simulink model "Bixler_withAutoPilot"  (R2018b)
settings: Solver=FixedStepAuto  StartTime=0.0  StopTime=inf  RelTol=1e-3
undefined symbols (not defined in the file or in its folder): dev, Main, pwm_output0
libraries: simulink x5, px4uORBlib x4, aerolibutil x3, px4Sensorslib x2, vrlib x1, px4lib x1, sharedtransform x1
(part 1 of 2)
settings Model: SimulationMode=external  ExtModeTrigDuration=10  Creator=Robert  LastModifiedBy=Robert
settings SolverCC: PositivePriorityOrder=on
settings DataIOCC: SaveState=on
settings OptimizationCC: DefaultUnderspecifiedDataType=single  EnhancedBackFolding=on  PassReuseOutputArgsAs=Individual arguments  MaxStackSize=64  OptimizeBlockOrder=speed  DifferentSizesBufferReuse=on  OptimizationCustomize=off
settings DebuggingCC: ParameterTunabilityLossMsg=error
settings HardwareCC: ProdBitPerPointer=32  ProdBitPerSizeT=32  ProdBitPerPtrDiffT=32  ProdLargestAtomicInteger=Long  ProdLargestAtomicFloat=Double  ProdWordSize=32  ProdLongLongMode=on  ProdHWDeviceType=ARM Compatible->ARM Cortex
settings SFSimCC: MATLABDynamicMemAlloc=off
settings RTWCC: SystemTargetFile=ert.tlc  HardwareBoard=PX4 Pixhawk 1  TLCOptions="-aInlineSetEventsForThisBaseRateFcn=TLC_FALSE -aSuppressMultiTaskScheduler=TLC_FALSE  -aRateBasedStepFcn=0"  TemplateMakefile=ert_default_tmf  GenerateReport=on  Toolchain=GNU Tools for PX4 Autopilots  IncludeHyperlinkInReport=on  LaunchReport=on  TargetLang=C++  GenerateTraceInfo=on  GenerateTraceReport=on  GenerateTraceReportSl=on  GenerateTraceReportSf=on  GenerateTraceReportEml=on
settings CodeAppCC: ForceParamTrailComments=on  IgnoreCustomStorageClasses=off  OperatorAnnotations=on  SimulinkDataObjDesc=on  SFDataObjDesc=on  InsertBlockDesc=on
settings ERTTargetCC: ExtMode=on  ExtModeMexArgs='127.0.0.1' 1 17725

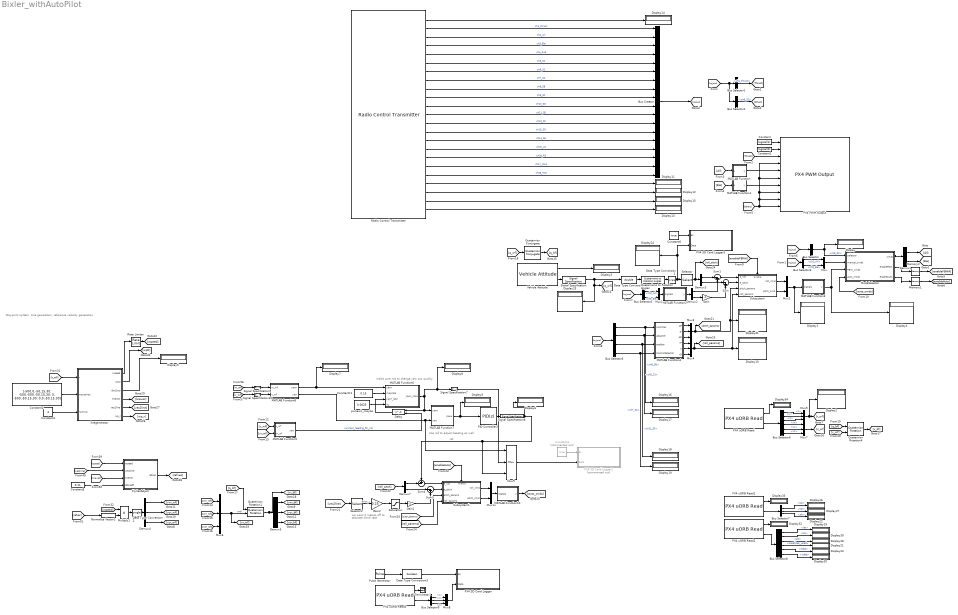
== system Bixler_withAutoPilot ==
  note: we want 4 metres off
      | to saturate climb rate
  note: Waypoint system,
      | Line generation,
      | reference velocity generation
  note: make sure not to change yaw too quickly
  note: Use roll to adjust heading as well
  Bus Creator : BusCreator  Inputs=18
  Bus Selector : BusSelector  OutputSignals=ch9_SC
  Bus Selector1 : BusSelector  OutputSignals=ch1_thrust
  Bus Selector2 : BusSelector  OutputSignals=ch6_S2
  Bus Selector3 : BusSelector  OutputSignals=ch2_Ail,ch3_Ele
  Bus Selector4 : BusSelector  OutputSignals=ch2_Ail,ch3_Ele
  Bus Selector5 : BusSelector  OutputSignals=ch8_SB,ch5_S1,ch12_SF,ch7_SA
  Bus Selector6 : BusSelector  OutputSignals=x,y,z,vx,vy,vz
  Bus Selector7 : BusSelector  OutputSignals=lat,lon,alt
  Bus Selector8 : BusSelector  OutputSignals=lat,lon,alt,satellites_used,hdop,vdop
  Bus Selector9 : BusSelector  OutputSignals=x,y,z
  Constant : Constant  Value=logical(1)
  Constant1 : Constant  Value=logical(0)
  Constant11 : Constant  Value=0.15  OutDataTypeStr=single
  Constant2 : Constant  Value=[-500,0,-50,15,30; -500,-500,-50,15,30; 0, -500,-50,15,30; 0,0,-50,15,30]  OutDataTypeStr=single
  Constant3 : Constant  Value=4  OutDataTypeStr=single
  Constant4 : Constant  Commented=on  Value=true  OutDataTypeStr=boolean
  Constant5 : Constant  Value=0.11  OutDataTypeStr=single  SampleTime=-1
  Constant6 : Constant  Value=true  OutDataTypeStr=boolean
  Data Type Conversion : DataTypeConversion  OutDataTypeStr=double
  Data Type Conversion1 : DataTypeConversion  OutDataTypeStr=single
  Data Type Conversion2 : DataTypeConversion  OutDataTypeStr=single
  Data Type Conversion3 : DataTypeConversion  OutDataTypeStr=boolean
  Delay : Delay  DelayLength=1  InitialConditionSource=Input port
      settings: InputPortMap=u0,p4
  Demux{1..3,7} (4 alike) : Demux  Outputs=2
  Demux4 : Demux  Outputs=3
  Demux5 : Demux  Outputs=3
  Display{,1..34} (35 alike) : Display
  FlyVecAdjust : MATLAB Function  TreatAsAtomicUnit=on
  Gain : Gain  Gain=-1
  Gain1 : Gain  Gain=-1
  Gain2 : Gain  Gain=0.25
  MATLAB Function : MATLAB Function  TreatAsAtomicUnit=on
  MATLAB Function1 : MATLAB Function  TreatAsAtomicUnit=on
  MATLAB Function10 : MATLAB Function  TreatAsAtomicUnit=on
  MATLAB Function2 : MATLAB Function  TreatAsAtomicUnit=on
  MATLAB Function3 : MATLAB Function  TreatAsAtomicUnit=on
  MATLAB Function4 : MATLAB Function  TreatAsAtomicUnit=on
  MATLAB Function5 : MATLAB Function  TreatAsAtomicUnit=on
  MATLAB Function6 : MATLAB Function  TreatAsAtomicUnit=on
  MATLAB Function7 : MATLAB Function  TreatAsAtomicUnit=on
  MATLAB Function8 : MATLAB Function  TreatAsAtomicUnit=on
  Memory1 : Memory
  Memory2 : Memory
  ModeSelector : MATLAB Function  TreatAsAtomicUnit=on
  Multiply1 : Product
  Mux{,1..2,10} (4 alike) : Mux  Inputs=2
  Mux{3..9} (7 alike) : Mux  Inputs=3
  Normalize Vector1 : vrlib/Utilities/Normalize Vector  maxzero=0
      settings: SourceProductName=Simulink 3D Animation  SourceProductBaseCode=VR
  PID Controller2 : simulink/Continuous/PID Controller  Controller=PID  Form=Parallel  TimeDomain=Discrete-time  SampleTime=-1  IntegratorMethod=Forward Euler  FilterMethod=Forward Euler  ControllerParametersSource=internal  P=1  I=0  D=0.5*0  UseFilter=off  N=100  TunerSelectOption=Transfer Function Based (PID Tuner App)  InitialConditionSource=internal  InitialConditionForIntegrator=0  InitialConditionForFilter=0  DifferentiatorICPrevScaledInput=0  ExternalReset=none  TrackingMode=off  Kt=1  LimitOutput=on  UpperSaturationLimit=deg2rad(30)  LowerSaturationLimit=-deg2rad(30)  LinearizeAsGain=on  AntiWindupMode=clamping  Kb=1  POutMin=[]  POutMax=[]  IOutMin=[]  IOutMax=[]  DOutMin=[]  DOutMax=[]  NOutMin=[]  NOutMax=[]  SumOutMin=[]  SumOutMax=[]  SaturationOutMin=[]  SaturationOutMax=[]  PParamMin=[]  PParamMax=[]  IParamMin=[]  IParamMax=[]  DParamMin=[]  DParamMax=[]  NParamMin=[]  NParamMax=[]  KbParamMin=[]  KbParamMax=[]  KtParamMin=[]  KtParamMax=[]  KbOutMin=[]  KbOutMax=[]  KtOutMin=[]  KtOutMax=[]  IntegratorOutMin=[]  IntegratorOutMax=[]  FilterOutMin=[]  FilterOutMax=[]  SumI1OutMin=[]  SumI1OutMax=[]  SumI2OutMin=[]  SumI2OutMax=[]  SumI3OutMin=[]  SumI3OutMax=[]  SumI4OutMin=[]  SumI4OutMax=[]  SumDOutMin=[]  SumDOutMax=[]  DifferentiatorOutMin=[]  DifferentiatorOutMax=[]  FilterDiffOutCoefMin=[]  FilterDiffOutCoefMax=[]  ReciprocalOutMin=[]  ReciprocalOutMax=[]  SumDenOutMin=[]  SumDenOutMax=[]  SumNumOutMin=[]  SumNumOutMax=[]  DivideOutMin=[]  DivideOutMax=[]  IntegratorContinuousStateAttributes=''  IntegratorStateMustResolveToSignalObject=off  IntegratorRTWStateStorageClass=Auto  FilterContinuousStateAttributes=''  FilterStateMustResolveToSignalObject=off  FilterRTWStateStorageClass=Auto  ParallelPVariant=InternalParameters  IdealPVariant=Disabled  IVariant=InternalParameters  DVariant=InternalParameters  IntegratorVariant=Discrete  SatVariant=Enabled  AWVariant=DiscClampingParallel  PCopyVariant=Disabled  TRVariant=Disabled  FdbkBlocksVariant=Forward  IdealPFdbkVariant=Disabled  SatFdbkVariant=Disabled  DerivativeFilterVariant=Differentiator  NVariant=Passthrough  NCopyVariant=Disabled_SignalSpec  FilterICVariant=InternalICsDifferentiator  IntegratorICVariant=InternalICs  ExternalResetVariant=Disabled  TRSumVariant=Passthrough  SumFdbkVariant=Disabled  SumVariant=Sum_PID
  PX4 PWM Output : px4lib/PX4 PWM Output  pwmDevice=Main (/dev/pwm_output0)  pwmChannel1_=on  pwmChannel2_=on  pwmChannel3_=on  pwmChannel4_=on  pwmChannel5_=on  pwmChannel6_=on  pwmChannel7_=on  pwmChannel8_=on  forceTerminateFailsafe=off  outputErrorStatus=off
      settings: SourceProductName=Embedded Coder Support Package for PX4 Autopilots
  PX4 SD Card Logger : Subsystem  mask(PX4 SD Card Logger){logfile=/fs/microsd/log, logfilename=accel_data, cacheflag=off, numRecs=100}
      mask prompts: logfile "Log Folder"; logfilename "Log File Name"; cacheflag "Cache in Memory"; numRecs "Maximum Record Count"
      mask help:
      | Log data to a specified file on the SD card
      |
      | The block accepts two inputs, enable and data. The incoming data is logged into the SD card when the enable signal is high and the number of data points logged is less than the Maximum Record Count specified.
      |
      | The specified folder should be present in the SD card for logging.
      |
      | If Cache in Memory is unchecked, the data is written to the SD card at every timestep.  If Cache in Memory is checked, data is cached in the memory and is written to SD card only when enable goes low or when the number of data points logged reaches the Maximum Record Count specified.
      mask init:
      | logname=uint8([logfile,'/',logfilename]);
      mask Help: eval('codertarget.internal.helpView(''px4'',''px4sdcardexample'')');
      mask Display:
      | fprintf([get_param(gcb,'logfile'),'/',get_param(gcb,'logfilename')])
      | port_label('input',1,'en')
      | port_label('input',2,'data')
  PX4 SD Card Logger1 : Subsystem  Commented=on  mask(PX4 SD Card Logger){logfile=/fs/microsd/log, logfilename=yaw_yawrs_rollr, cacheflag=off, numRecs=100}
      mask prompts: logfile "Log Folder"; logfilename "Log File Name"; cacheflag "Cache in Memory"; numRecs "Maximum Record Count"
      mask help:
      | Log data to a specified file on the SD card
      |
      | The block accepts two inputs, enable and data. The incoming data is logged into the SD card when the enable signal is high and the number of data points logged is less than the Maximum Record Count specified.
      |
      | The specified folder should be present in the SD card for logging.
      |
      | If Cache in Memory is unchecked, the data is written to the SD card at every timestep.  If Cache in Memory is checked, data is cached in the memory and is written to SD card only when enable goes low or when the number of data points logged reaches the Maximum Record Count specified.
      mask init:
      | logname=uint8([logfile,'/',logfilename]);
      mask Help: eval('codertarget.internal.helpView(''px4'',''px4sdcardexample'')');
      mask Display:
      | fprintf([get_param(gcb,'logfile'),'/',get_param(gcb,'logfilename')])
      | port_label('input',1,'en')
      | port_label('input',2,'data')
  PX4 SD Card Logger3 : Subsystem  mask(PX4 SD Card Logger){logfile=/fs/microsd/log, logfilename=YPR, cacheflag=off, numRecs=10000}
      mask prompts: logfile "Log Folder"; logfilename "Log File Name"; cacheflag "Cache in Memory"; numRecs "Maximum Record Count"
      mask help:
      | Log data to a specified file on the SD card
      |
      | The block accepts two inputs, enable and data. The incoming data is logged into the SD card when the enable signal is high and the number of data points logged is less than the Maximum Record Count specified.
      |
      | The specified folder should be present in the SD card for logging.
      |
      | If Cache in Memory is unchecked, the data is written to the SD card at every timestep.  If Cache in Memory is checked, data is cached in the memory and is written to SD card only when enable goes low or when the number of data points logged reaches the Maximum Record Count specified.
      mask init:
      | logname=uint8([logfile,'/',logfilename]);
      mask Help: eval('codertarget.internal.helpView(''px4'',''px4sdcardexample'')');
      mask Display:
      | fprintf([get_param(gcb,'logfile'),'/',get_param(gcb,'logfilename')])
      | port_label('input',1,'en')
      | port_label('input',2,'data')
  PX4 uORB Read : px4uORBlib/PX4 uORB Read  uORBTopic=vehicle_local_position  sampleTime=0.001  BlockingMode=off  BlockTimeout=1e-3
      settings: SourceProductName=Embedded Coder Support Package for PX4 Autopilots
  PX4 uORB Read1 : px4uORBlib/PX4 uORB Read  uORBTopic=vehicle_global_position  sampleTime=0.001  BlockingMode=off  BlockTimeout=1e-3
      settings: SourceProductName=Embedded Coder Support Package for PX4 Autopilots
  PX4 uORB Read2 : px4uORBlib/PX4 uORB Read  uORBTopic=vehicle_gps_position  sampleTime=0.001  BlockingMode=off  BlockTimeout=1e-3
      settings: SourceProductName=Embedded Coder Support Package for PX4 Autopilots
  PX4 uORB Read3 : px4uORBlib/PX4 uORB Read  uORBTopic=vehicle_local_position  sampleTime=-1  BlockingMode=off  BlockTimeout=1e-3
      settings: SourceProductName=Embedded Coder Support Package for PX4 Autopilots
  Pulse Generator : DiscretePulseGenerator  Period=50  PulseWidth=20  SampleTime=0.01  VectorParams1D=off
  Quaternion Conjugate : aerolibutil/Quaternion Conjugate
      settings: SourceProductName=Aerospace Blockset  SourceProductBaseCode=AE
  Quaternion Rotation1 : aerolibutil/Quaternion Rotation
  Quaternion Rotation4 : aerolibutil/Quaternion Rotation
  Quaternions to Rotation Angles : sharedtransform/Quaternions to Rotation Angles  rotationOrder=ZYX  aMode=aMode
      settings: SourceProductBaseCode=AE
  Radio Control Transmitter : px4Sensorslib/Radio Control Transmitter  channel1=on  channel2=on  channel3=on  channel4=on  channel5=on  channel6=on  channel7=on  channel8=on  channel9=on  channel10=on  channel11=on  channel12=on  channel13=on  channel14=on  channel15=on  channel16=on  channel17=on  channel18=on  channel_count=on  rssi=on  rc_input_source=on  timestamp_last_signal=on  time_stamp=off  sampleTime=1/250  BlockingMode=off  BlockTimeout=5
      settings: SourceProductName=Embedded Coder Support Package for PX4 Autopilots
  Rate Limiter : RateLimiter  SampleTimeMode=inherited  InitialCondition=0.01
  Saturation : Saturate  UpperLimit=deg2rad(15)  LowerLimit=deg2rad(-20)
  Selector : Selector  InputPortWidth=3  IndexOptions=Index vector (dialog)  Indices=[3 2]  OutputSizes=1
  Selector2 : Selector  InputPortWidth=3  IndexOptions=Index vector (dialog)  Indices=[3]  OutputSizes=1
  Signal Specification : SignalSpecification  OutDataTypeStr=single
  Signal Specification10 : SignalSpecification  OutDataTypeStr=single  Dimensions=3
  Signal Specification7 : SignalSpecification  OutDataTypeStr=single  Dimensions=1
  Signal Specification8 : SignalSpecification  OutDataTypeStr=single  Dimensions=1
  Signal Specification9 : SignalSpecification  OutDataTypeStr=single  Dimensions=3
  Subsystem : Subsystem
  Subsystem1 : Subsystem
  Sum : Sum  Inputs=|-+
  Sum1 : Sum  Inputs=|-+
  Sum3 : Sum  Inputs=|-+
  Sum4 : Sum  Inputs=+-|
  Terminator1 : Terminator
  Vehicle Attitude : px4Sensorslib/Vehicle Attitude  rollRate=off  pitchRate=off  yawRate=off  quaternion=on  uorbTimeStamp=off  BlockingMode=off  BlockTimeout=0.001  sampleTime=1/250
      settings: SourceProductName=Embedded Coder Support Package for PX4 Autopilots
  linegenerator : MATLAB Function  TreatAsAtomicUnit=on
  "pixhawk_maybe " : Constant  Value=0.0025  OutDataTypeStr=single
  wires:
  Vehicle Attitude/2 -> Signal Specification/1
  Vehicle Attitude/1 -> Display3/1
  Radio Control Transmitter/8 -> Bus Creator/7  "ch7_SA"
  Radio Control Transmitter/7 -> Bus Creator/6  "ch6_S2"
  Radio Control Transmitter/6 -> Bus Creator/5  "ch5_S1"
  Radio Control Transmitter/2 -> Bus Creator/1  "ch1_thrust"
  Radio Control Transmitter/3 -> Bus Creator/2  "ch2_Ail"
  Radio Control Transmitter/4 -> Bus Creator/3  "ch3_Ele"
  Radio Control Transmitter/5 -> Bus Creator/4  "ch4_Rud"
  Radio Control Transmitter/9 -> Bus Creator/8  "ch8_SB"
  Radio Control Transmitter/20 -> Display11/1
  Radio Control Transmitter/21 -> Display12/1
  Radio Control Transmitter/23 -> Display13/1
  Radio Control Transmitter/1 -> Display14/1
  Radio Control Transmitter/22 -> Display15/1
  Constant/1 -> PX4 PWM Output/1
  Bus Selector1/1 -> [Thrust]  "<ch1_thrust>"
  [Others] -> PX4 PWM Output/6, PX4 PWM Output/4, PX4 PWM Output/8, PX4 PWM Output/9, PX4 PWM Output/10
  Constant1/1 -> PX4 PWM Output/2
  Bus Creator/1 -> [rc_bus]
  Quaternions to Rotation Angles/1 -> Data Type Conversion1/1
  Bus Selector/1 -> ModeSelector/1(selector), Display/1  "<ch9_SC>"
  Demux3/1 -> Sum1/1
  Demux3/2 -> Sum/1
  Mux2/1 -> Display1/1, MATLAB Function3/1(signals)
  Signal Specification/1 -> [q_wf], Display25/1, Data Type Conversion/1
  [rc_bus] -> Bus Selector2/1, Bus Selector1/1
  [Thrust] -> PX4 PWM Output/3
  [Ail] -> MATLAB Function/1(u)
  [Ele] -> MATLAB Function1/1(u)
  [rc_bus] -> Bus Selector3/1
  [rc_bus] -> Bus Selector/1
  MATLAB Function3/1(y) -> ModeSelector/3(FBW_cmds), Display4/1
  Bus Selector3/1 -> Mux/1  "<ch2_Ail>"
  Bus Selector3/2 -> Mux/2  "<ch3_Ele>"
  Mux/1 -> ModeSelector/2(manual_cmds)
  ModeSelector/1(cmds) -> Demux1/1
  Demux1/1 -> [Ail]
  Demux1/2 -> [Ele]
  Bus Selector2/1 -> [Others]  "<ch6_S2>"
  Data Type Conversion/1 -> Quaternions to Rotation Angles/1
  MATLAB Function/1(y) -> PX4 PWM Output/5
  MATLAB Function1/1(y) -> PX4 PWM Output/7
  Demux2/2 -> Gain/1
  [rc_bus] -> Bus Selector4/1
  Bus Selector4/1 -> Mux1/1  "<ch2_Ail>"
  Bus Selector4/2 -> Mux1/2  "<ch3_Ele>"
  Mux1/1 -> MATLAB Function2/1(signals)
  MATLAB Function2/1(y) -> Demux2/1
  Demux2/1 -> Sum1/2
  Mux4/1 -> [roll_params], Subsystem/4(roll_params), Display10/1
  [rc_bus] -> Bus Selector5/1
  Bus Selector5/2 -> Display17/1, MATLAB Function4/2(adjuster)  "<ch5_S1>"
  Bus Selector5/1 -> Display16/1, MATLAB Function4/1(switcher)  "<ch8_SB>"
  MATLAB Function4/1(pP) -> Mux3/1
  MATLAB Function4/2(pI) -> Mux3/2
  MATLAB Function4/3(pD) -> Mux3/3
  Bus Selector5/3 -> Display18/1, MATLAB Function4/3(enabler)  "<ch12_SF>"
  Radio Control Transmitter/10 -> Bus Creator/9  "ch9_SC"
  Radio Control Transmitter/11 -> Bus Creator/10  "ch10_SD"
  Radio Control Transmitter/12 -> Bus Creator/11  "ch11_SE"
  Radio Control Transmitter/13 -> Bus Creator/12  "ch12_SF"
  Radio Control Transmitter/14 -> Bus Creator/13  "ch13_SG"
  Radio Control Transmitter/15 -> Bus Creator/14  "ch14_SH"
  Radio Control Transmitter/16 -> Bus Creator/15  "ch15_LS"
  Radio Control Transmitter/17 -> Bus Creator/16  "ch16_RS"
  Radio Control Transmitter/18 -> Bus Creator/17  "ch17_MAX"
  Radio Control Transmitter/19 -> Bus Creator/18  "ch18_MIN"
  MATLAB Function4/4(rP) -> Mux4/1
  MATLAB Function4/5(rI) -> Mux4/2
  MATLAB Function4/6(rD) -> Mux4/3
  Bus Selector5/4 -> Display19/1, MATLAB Function4/4(ControlSelector)  "<ch7_SA>"
  PX4 uORB Read/2 -> Bus Selector6/1
  PX4 uORB Read1/2 -> Bus Selector7/1
  PX4 uORB Read2/2 -> Bus Selector8/1
  PX4 uORB Read/1 -> Display34/1
  PX4 uORB Read1/1 -> Display33/1
  PX4 uORB Read2/1 -> Display32/1
  Bus Selector6/1 -> Mux5/1  "<x>"
  Bus Selector6/2 -> Mux5/2  "<y>"
  Bus Selector6/3 -> Mux5/3  "<z>"
  Bus Selector7/1 -> Display26/1  "<lat>"
  Bus Selector7/2 -> Display27/1  "<lon>"
  Bus Selector7/3 -> Display22/1  "<alt>"
  Bus Selector8/1 -> Display29/1  "<lat>"
  Bus Selector8/2 -> Display30/1  "<lon>"
  Bus Selector8/3 -> Display28/1  "<alt>"
  Sum1/1 -> Subsystem/1(e_roll)
  Sum/1 -> Subsystem/2(e_pitch)
  Subsystem/1(roll_cmd) -> Mux2/1
  Subsystem/2(pitch_cmd) -> Mux2/2
  [enableFBWA] -> Subsystem/Enable
  Gain/1 -> Sum/2
  Mux3/1 -> [pitch_params], Subsystem/3(pitch_params), Display31/1
  ModeSelector/2(enableFBW) -> Memory2/1
  Selector/1 -> [roll_pitch], Demux3/1
  ModeSelector/3(enableAuto) -> Memory1/1
  Memory1/1 -> [enableAuto]
  Memory2/1 -> [enableFBWA]
  Mux5/1 -> Display2/1, [r_wf]
  [rspeed] -> Multiply1/1
  linegenerator/1(rspeed) -> Rate Limiter/1
  linegenerator/2(wpN) -> [wpN]
  linegenerator/4(linevec) -> [linevec]
  Constant5/1 -> FlyVecAdjust/4(d2lcoeff)
  [linevec] -> FlyVecAdjust/3(linevec)
  [refvec] -> Normalize Vector1/1
  [vec2line] -> FlyVecAdjust/2(vec2line)
  Normalize Vector1/1 -> Multiply1/2
  linegenerator/6(wp_r) -> [wp_r]
  Rate Limiter/1 -> [rspeed]
  Demux4/1 -> [vxr_wf]
  FlyVecAdjust/1(refvec) -> [refvec]
  Demux4/2 -> [vyr_wf]
  Demux4/3 -> [vzr_wf]
  linegenerator/5(vec2line) -> [vec2line]
  [rspeed] -> FlyVecAdjust/1(rspeed)
  Multiply1/1 -> Data Type Conversion2/1
  [v_wf] -> MATLAB Function5/1(v_wf)
  [vr_wf] -> MATLAB Function5/2(vr_wf)
  [r_wf] -> linegenerator/1(r)
  linegenerator/3(dist2wp) -> Display5/1
  [vzr_wf] -> Mux6/3
  [vyr_wf] -> Mux6/2
  [vxr_wf] -> Mux6/1
  Demux5/2 -> [vyr_bf]
  Demux5/3 -> [vzr_bf]
  Demux5/1 -> [vxr_bf]
  Quaternion Rotation1/1 -> Demux5/1, [vr_bf]
  [q_bf] -> Quaternion Rotation1/1
  Mux6/1 -> [vr_wf], Quaternion Rotation1/2  "vref"
  [q_wf] -> Quaternion Conjugate/1
  Quaternion Conjugate/1 -> [q_bf]
  Bus Selector6/4 -> Mux7/1  "<vx>"
  Bus Selector6/5 -> Mux7/2  "<vy>"
  Bus Selector6/6 -> Mux7/3  "<vz>"
  Mux7/1 -> [v_wf]
  Quaternion Rotation4/1 -> [v_bf]
  [v_wf] -> Quaternion Rotation4/2
  [q_bf] -> Quaternion Rotation4/1
  [auto_cmds] -> ModeSelector/4(auto_cmds)
  MATLAB Function5/1(yaw) -> Delay/2  "currrent_heading_for_init"
  [vr_wf] -> Signal Specification9/1
  PID Controller2/1 -> Signal Specification8/1
  Delay/1 -> MATLAB Function6/3(yawr_last)
  [v_wf] -> Signal Specification10/1
  MATLAB Function8/2(yaw) -> Mux9/1, MATLAB Function7/2(yaw)
  Signal Specification9/1 -> MATLAB Function8/1(vr_wf)
  MATLAB Function8/1(yawr) -> Display7/1, MATLAB Function6/1(yawr)
  Signal Specification8/1 -> Display6/1, Mux9/3, Sum4/1  "roll"
  MATLAB Function7/1(yawe) -> Display9/1, PID Controller2/1
  Signal Specification10/1 -> MATLAB Function8/2(v_wf)
  Constant11/1 -> MATLAB Function6/2(maxrate)
  MATLAB Function6/1(yawr_slow) -> Display8/1, Signal Specification7/1, Delay/1, MATLAB Function7/1(yawr)
  Signal Specification7/1 -> Mux9/2
  [vec2line] -> Selector2/1
  Selector2/1 -> Gain2/1  "error_z"
  Subsystem1/1(roll_cmd) -> Mux10/1
  Gain1/1 -> Sum3/2
  Subsystem1/2(pitch_cmd) -> Mux10/2
  Sum4/1 -> Subsystem1/1(e_roll)
  Sum3/1 -> Subsystem1/2(e_pitch)
  [enableAuto] -> Subsystem1/Enable
  Gain2/1 -> Saturation/1
  Demux7/2 -> Sum3/1
  Demux7/1 -> Sum4/2
  [pitch_params] -> Subsystem1/3(pitch_params)
  [roll_params] -> Subsystem1/4(roll_params)
  [roll_pitch] -> Demux7/1
  Mux10/1 -> MATLAB Function10/1(signals)
  MATLAB Function10/1(y) -> [auto_cmds]
  "pixhawk_maybe "/1 -> MATLAB Function6/4(Ts)
  Constant2/1 -> linegenerator/2(waypoints)
  Constant3/1 -> linegenerator/3(numwp)
  Data Type Conversion2/1 -> Demux4/1
  Saturation/1 -> Gain1/1
  PX4 uORB Read3/2 -> Bus Selector9/1
  Bus Selector9/1 -> Mux8/1  "<x>"
  Mux8/1 -> PX4 SD Card Logger/2(Data)
  PX4 uORB Read3/1 -> Terminator1/1
  Bus Selector9/2 -> Mux8/2  "<y>"
  Data Type Conversion3/1 -> PX4 SD Card Logger/1(En)
  Bus Selector9/3 -> Mux8/3  "<z>"
  Pulse Generator/1 -> Data Type Conversion3/1
  Mux9/1 -> PX4 SD Card Logger1/2(Data)
  Bus Selector8/4 -> Display21/1  "<satellites_used>"
  Bus Selector8/5 -> Display23/1  "<hdop>"
  Bus Selector8/6 -> Display20/1  "<vdop>"
  Constant4/1 -> PX4 SD Card Logger1/1(En)
  Constant6/1 -> PX4 SD Card Logger3/1(En)
  Data Type Conversion1/1 -> Display24/1, PX4 SD Card Logger3/2(Data), Selector/1

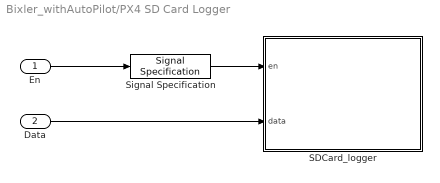
== system Bixler_withAutoPilot/PX4 SD Card Logger ==
  En : Inport
  Data : Inport  Port=2
  SDCard_logger : MATLAB Function  TreatAsAtomicUnit=on
  Signal Specification : SignalSpecification  OutDataTypeStr=boolean
  wires:
  Signal Specification/1 -> SDCard_logger/1(en)
  En/1 -> Signal Specification/1
  Data/1 -> SDCard_logger/2(data)

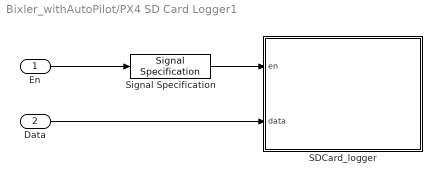
== system Bixler_withAutoPilot/PX4 SD Card Logger1 ==
  En : Inport
  Data : Inport  Port=2
  SDCard_logger : MATLAB Function  TreatAsAtomicUnit=on
  Signal Specification : SignalSpecification  OutDataTypeStr=boolean
  wires:
  Signal Specification/1 -> SDCard_logger/1(en)
  En/1 -> Signal Specification/1
  Data/1 -> SDCard_logger/2(data)

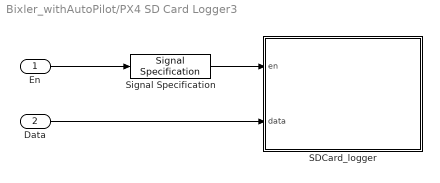
== system Bixler_withAutoPilot/PX4 SD Card Logger3 ==
  En : Inport
  Data : Inport  Port=2
  SDCard_logger : MATLAB Function  TreatAsAtomicUnit=on
  Signal Specification : SignalSpecification  OutDataTypeStr=boolean
  wires:
  Signal Specification/1 -> SDCard_logger/1(en)
  En/1 -> Signal Specification/1
  Data/1 -> SDCard_logger/2(data)

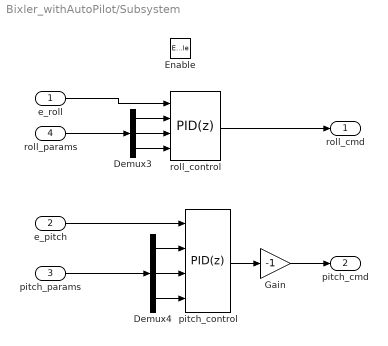
== system Bixler_withAutoPilot/Subsystem ==
  e_roll : Inport
  e_pitch : Inport  Port=2
  pitch_params : Inport  Port=3
  roll_params : Inport  Port=4
  Enable : EnablePort
  Demux3 : Demux  Outputs=3
  Demux4 : Demux  Outputs=3
  Gain : Gain  Gain=-1
  pitch_control : simulink/Continuous/PID Controller  Controller=PID  Form=Parallel  TimeDomain=Discrete-time  SampleTime=1/250  IntegratorMethod=Backward Euler  FilterMethod=Forward Euler  ControllerParametersSource=external  P=1  I=0  D=0  UseFilter=off  N=100  TunerSelectOption=Transfer Function Based (PID Tuner App)  InitialConditionSource=internal  InitialConditionForIntegrator=0  InitialConditionForFilter=0  DifferentiatorICPrevScaledInput=0  ExternalReset=none  TrackingMode=off  Kt=1  LimitOutput=on  UpperSaturationLimit=1  LowerSaturationLimit=-1  LinearizeAsGain=off  AntiWindupMode=clamping  Kb=1  PGainOutDataTypeStr=single  PProdOutDataTypeStr=single  POutMin=[]  POutMax=[]  IGainOutDataTypeStr=single  IProdOutDataTypeStr=single  IOutMin=[]  IOutMax=[]  DGainOutDataTypeStr=single  DProdOutDataTypeStr=single  DOutMin=[]  DOutMax=[]  NOutMin=[]  NOutMax=[]  SumOutDataTypeStr=single  SumOutMin=[]  SumOutMax=[]  SaturationOutDataTypeStr=single  SaturationOutMin=[]  SaturationOutMax=[]  PParamDataTypeStr=single  PParamMin=[]  PParamMax=[]  IParamDataTypeStr=single  IParamMin=[]  IParamMax=[]  DParamDataTypeStr=single  DParamMin=[]  DParamMax=[]  NParamMin=[]  NParamMax=[]  KbParamMin=[]  KbParamMax=[]  KtParamMin=[]  KtParamMax=[]  KbOutMin=[]  KbOutMax=[]  KtOutMin=[]  KtOutMax=[]  IntegratorOutDataTypeStr=single  IntegratorOutMin=[]  IntegratorOutMax=[]  FilterOutMin=[]  FilterOutMax=[]  SumI1OutMin=[]  SumI1OutMax=[]  SumI2OutMin=[]  SumI2OutMax=[]  SumI3OutMin=[]  SumI3OutMax=[]  SumI4OutMin=[]  SumI4OutMax=[]  SumDOutMin=[]  SumDOutMax=[]  SumAccumDataTypeStr=single  DifferentiatorOutDataTypeStr=single  DifferentiatorOutMin=[]  DifferentiatorOutMax=[]  FilterDiffOutCoefMin=[]  FilterDiffOutCoefMax=[]  ReciprocalOutMin=[]  ReciprocalOutMax=[]  SumDenOutMin=[]  SumDenOutMax=[]  SumNumOutMin=[]  SumNumOutMax=[]  DivideOutMin=[]  DivideOutMax=[]  IntegratorContinuousStateAttributes=''  IntegratorStateMustResolveToSignalObject=off  IntegratorRTWStateStorageClass=Auto  FilterContinuousStateAttributes=''  FilterStateMustResolveToSignalObject=off  FilterRTWStateStorageClass=Auto  ParallelPVariant=ExternalParameters  IdealPVariant=Disabled  IVariant=ExternalParameters  DVariant=ExternalParameters  IntegratorVariant=Discrete  SatVariant=Enabled  AWVariant=DiscClampingParallel  PCopyVariant=Disabled  TRVariant=Disabled  FdbkBlocksVariant=Feedback  IdealPFdbkVariant=Passthrough  SatFdbkVariant=Passthrough  DerivativeFilterVariant=Differentiator  NVariant=Passthrough  NCopyVariant=Disabled_SignalSpec  FilterICVariant=InternalICsDifferentiator  IntegratorICVariant=InternalICs  ExternalResetVariant=Disabled  TRSumVariant=Passthrough  SumFdbkVariant=Enabled  SumVariant=Sum_PID
  roll_control : simulink/Continuous/PID Controller  Controller=PID  Form=Parallel  TimeDomain=Discrete-time  SampleTime=1/250  IntegratorMethod=Backward Euler  FilterMethod=Forward Euler  ControllerParametersSource=external  P=1  I=0  D=0  UseFilter=off  N=100  TunerSelectOption=Transfer Function Based (PID Tuner App)  InitialConditionSource=internal  InitialConditionForIntegrator=0  InitialConditionForFilter=0  DifferentiatorICPrevScaledInput=0  ExternalReset=none  TrackingMode=off  Kt=1  LimitOutput=on  UpperSaturationLimit=1  LowerSaturationLimit=-1  LinearizeAsGain=off  AntiWindupMode=clamping  Kb=1  PGainOutDataTypeStr=single  PProdOutDataTypeStr=single  POutMin=[]  POutMax=[]  IGainOutDataTypeStr=single  IProdOutDataTypeStr=single  IOutMin=[]  IOutMax=[]  DGainOutDataTypeStr=single  DProdOutDataTypeStr=single  DOutMin=[]  DOutMax=[]  NOutMin=[]  NOutMax=[]  SumOutDataTypeStr=single  SumOutMin=[]  SumOutMax=[]  SaturationOutDataTypeStr=single  SaturationOutMin=[]  SaturationOutMax=[]  PParamDataTypeStr=single  PParamMin=[]  PParamMax=[]  IParamDataTypeStr=single  IParamMin=[]  IParamMax=[]  DParamDataTypeStr=single  DParamMin=[]  DParamMax=[]  NParamMin=[]  NParamMax=[]  KbParamMin=[]  KbParamMax=[]  KtParamMin=[]  KtParamMax=[]  KbOutMin=[]  KbOutMax=[]  KtOutMin=[]  KtOutMax=[]  IntegratorOutDataTypeStr=single  IntegratorOutMin=[]  IntegratorOutMax=[]  FilterOutMin=[]  FilterOutMax=[]  SumI1OutMin=[]  SumI1OutMax=[]  SumI2OutMin=[]  SumI2OutMax=[]  SumI3OutMin=[]  SumI3OutMax=[]  SumI4OutMin=[]  SumI4OutMax=[]  SumDOutMin=[]  SumDOutMax=[]  SumAccumDataTypeStr=single  DifferentiatorOutDataTypeStr=single  DifferentiatorOutMin=[]  DifferentiatorOutMax=[]  FilterDiffOutCoefMin=[]  FilterDiffOutCoefMax=[]  ReciprocalOutMin=[]  ReciprocalOutMax=[]  SumDenOutMin=[]  SumDenOutMax=[]  SumNumOutMin=[]  SumNumOutMax=[]  DivideOutMin=[]  DivideOutMax=[]  IntegratorContinuousStateAttributes=''  IntegratorStateMustResolveToSignalObject=off  IntegratorRTWStateStorageClass=Auto  FilterContinuousStateAttributes=''  FilterStateMustResolveToSignalObject=off  FilterRTWStateStorageClass=Auto  ParallelPVariant=ExternalParameters  IdealPVariant=Disabled  IVariant=ExternalParameters  DVariant=ExternalParameters  IntegratorVariant=Discrete  SatVariant=Enabled  AWVariant=DiscClampingParallel  PCopyVariant=Disabled  TRVariant=Disabled  FdbkBlocksVariant=Feedback  IdealPFdbkVariant=Passthrough  SatFdbkVariant=Passthrough  DerivativeFilterVariant=Differentiator  NVariant=Passthrough  NCopyVariant=Disabled_SignalSpec  FilterICVariant=InternalICsDifferentiator  IntegratorICVariant=InternalICs  ExternalResetVariant=Disabled  TRSumVariant=Passthrough  SumFdbkVariant=Enabled  SumVariant=Sum_PID
  roll_cmd : Outport
  pitch_cmd : Outport  Port=2
  wires:
  roll_control/1 -> roll_cmd/1
  Demux4/3 -> pitch_control/4
  Demux4/2 -> pitch_control/3
  Demux4/1 -> pitch_control/2
  pitch_params/1 -> Demux4/1
  Demux3/3 -> roll_control/4
  Demux3/2 -> roll_control/3
  Demux3/1 -> roll_control/2
  pitch_control/1 -> Gain/1
  e_roll/1 -> roll_control/1
  e_pitch/1 -> pitch_control/1
  roll_params/1 -> Demux3/1
  Gain/1 -> pitch_cmd/1

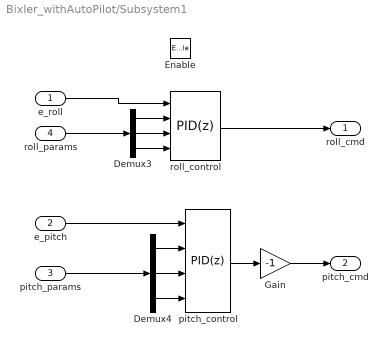
== system Bixler_withAutoPilot/Subsystem1 ==
  e_roll : Inport
  e_pitch : Inport  Port=2
  pitch_params : Inport  Port=3
  roll_params : Inport  Port=4
  Enable : EnablePort
  Demux3 : Demux  Outputs=3
  Demux4 : Demux  Outputs=3
  Gain : Gain  Gain=-1
  pitch_control : simulink/Continuous/PID Controller  Controller=PID  Form=Parallel  TimeDomain=Discrete-time  SampleTime=1/250  IntegratorMethod=Backward Euler  FilterMethod=Forward Euler  ControllerParametersSource=external  P=1  I=0  D=0  UseFilter=off  N=100  TunerSelectOption=Transfer Function Based (PID Tuner App)  InitialConditionSource=internal  InitialConditionForIntegrator=0  InitialConditionForFilter=0  DifferentiatorICPrevScaledInput=0  ExternalReset=none  TrackingMode=off  Kt=1  LimitOutput=on  UpperSaturationLimit=1  LowerSaturationLimit=-1  LinearizeAsGain=off  AntiWindupMode=clamping  Kb=1  PGainOutDataTypeStr=single  PProdOutDataTypeStr=single  POutMin=[]  POutMax=[]  IGainOutDataTypeStr=single  IProdOutDataTypeStr=single  IOutMin=[]  IOutMax=[]  DGainOutDataTypeStr=single  DProdOutDataTypeStr=single  DOutMin=[]  DOutMax=[]  NOutMin=[]  NOutMax=[]  SumOutDataTypeStr=single  SumOutMin=[]  SumOutMax=[]  SaturationOutDataTypeStr=single  SaturationOutMin=[]  SaturationOutMax=[]  PParamDataTypeStr=single  PParamMin=[]  PParamMax=[]  IParamDataTypeStr=single  IParamMin=[]  IParamMax=[]  DParamDataTypeStr=single  DParamMin=[]  DParamMax=[]  NParamMin=[]  NParamMax=[]  KbParamMin=[]  KbParamMax=[]  KtParamMin=[]  KtParamMax=[]  KbOutMin=[]  KbOutMax=[]  KtOutMin=[]  KtOutMax=[]  IntegratorOutDataTypeStr=single  IntegratorOutMin=[]  IntegratorOutMax=[]  FilterOutMin=[]  FilterOutMax=[]  SumI1OutMin=[]  SumI1OutMax=[]  SumI2OutMin=[]  SumI2OutMax=[]  SumI3OutMin=[]  SumI3OutMax=[]  SumI4OutMin=[]  SumI4OutMax=[]  SumDOutMin=[]  SumDOutMax=[]  SumAccumDataTypeStr=single  DifferentiatorOutDataTypeStr=single  DifferentiatorOutMin=[]  DifferentiatorOutMax=[]  FilterDiffOutCoefMin=[]  FilterDiffOutCoefMax=[]  ReciprocalOutMin=[]  ReciprocalOutMax=[]  SumDenOutMin=[]  SumDenOutMax=[]  SumNumOutMin=[]  SumNumOutMax=[]  DivideOutMin=[]  DivideOutMax=[]  IntegratorContinuousStateAttributes=''  IntegratorStateMustResolveToSignalObject=off  IntegratorRTWStateStorageClass=Auto  FilterContinuousStateAttributes=''  FilterStateMustResolveToSignalObject=off  FilterRTWStateStorageClass=Auto  ParallelPVariant=ExternalParameters  IdealPVariant=Disabled  IVariant=ExternalParameters  DVariant=ExternalParameters  IntegratorVariant=Discrete  SatVariant=Enabled  AWVariant=DiscClampingParallel  PCopyVariant=Disabled  TRVariant=Disabled  FdbkBlocksVariant=Feedback  IdealPFdbkVariant=Passthrough  SatFdbkVariant=Passthrough  DerivativeFilterVariant=Differentiator  NVariant=Passthrough  NCopyVariant=Disabled_SignalSpec  FilterICVariant=InternalICsDifferentiator  IntegratorICVariant=InternalICs  ExternalResetVariant=Disabled  TRSumVariant=Passthrough  SumFdbkVariant=Enabled  SumVariant=Sum_PID
  roll_control : simulink/Continuous/PID Controller  Controller=PID  Form=Parallel  TimeDomain=Discrete-time  SampleTime=1/250  IntegratorMethod=Backward Euler  FilterMethod=Forward Euler  ControllerParametersSource=external  P=1  I=0  D=0  UseFilter=off  N=100  TunerSelectOption=Transfer Function Based (PID Tuner App)  InitialConditionSource=internal  InitialConditionForIntegrator=0  InitialConditionForFilter=0  DifferentiatorICPrevScaledInput=0  ExternalReset=none  TrackingMode=off  Kt=1  LimitOutput=on  UpperSaturationLimit=1  LowerSaturationLimit=-1  LinearizeAsGain=off  AntiWindupMode=clamping  Kb=1  PGainOutDataTypeStr=single  PProdOutDataTypeStr=single  POutMin=[]  POutMax=[]  IGainOutDataTypeStr=single  IProdOutDataTypeStr=single  IOutMin=[]  IOutMax=[]  DGainOutDataTypeStr=single  DProdOutDataTypeStr=single  DOutMin=[]  DOutMax=[]  NOutMin=[]  NOutMax=[]  SumOutDataTypeStr=single  SumOutMin=[]  SumOutMax=[]  SaturationOutDataTypeStr=single  SaturationOutMin=[]  SaturationOutMax=[]  PParamDataTypeStr=single  PParamMin=[]  PParamMax=[]  IParamDataTypeStr=single  IParamMin=[]  IParamMax=[]  DParamDataTypeStr=single  DParamMin=[]  DParamMax=[]  NParamMin=[]  NParamMax=[]  KbParamMin=[]  KbParamMax=[]  KtParamMin=[]  KtParamMax=[]  KbOutMin=[]  KbOutMax=[]  KtOutMin=[]  KtOutMax=[]  IntegratorOutDataTypeStr=single  IntegratorOutMin=[]  IntegratorOutMax=[]  FilterOutMin=[]  FilterOutMax=[]  SumI1OutMin=[]  SumI1OutMax=[]  SumI2OutMin=[]  SumI2OutMax=[]  SumI3OutMin=[]  SumI3OutMax=[]  SumI4OutMin=[]  SumI4OutMax=[]  SumDOutMin=[]  SumDOutMax=[]  SumAccumDataTypeStr=single  DifferentiatorOutDataTypeStr=single  DifferentiatorOutMin=[]  DifferentiatorOutMax=[]  FilterDiffOutCoefMin=[]  FilterDiffOutCoefMax=[]  ReciprocalOutMin=[]  ReciprocalOutMax=[]  SumDenOutMin=[]  SumDenOutMax=[]  SumNumOutMin=[]  SumNumOutMax=[]  DivideOutMin=[]  DivideOutMax=[]  IntegratorContinuousStateAttributes=''  IntegratorStateMustResolveToSignalObject=off  IntegratorRTWStateStorageClass=Auto  FilterContinuousStateAttributes=''  FilterStateMustResolveToSignalObject=off  FilterRTWStateStorageClass=Auto  ParallelPVariant=ExternalParameters  IdealPVariant=Disabled  IVariant=ExternalParameters  DVariant=ExternalParameters  IntegratorVariant=Discrete  SatVariant=Enabled  AWVariant=DiscClampingParallel  PCopyVariant=Disabled  TRVariant=Disabled  FdbkBlocksVariant=Feedback  IdealPFdbkVariant=Passthrough  SatFdbkVariant=Passthrough  DerivativeFilterVariant=Differentiator  NVariant=Passthrough  NCopyVariant=Disabled_SignalSpec  FilterICVariant=InternalICsDifferentiator  IntegratorICVariant=InternalICs  ExternalResetVariant=Disabled  TRSumVariant=Passthrough  SumFdbkVariant=Enabled  SumVariant=Sum_PID
  roll_cmd : Outport
  pitch_cmd : Outport  Port=2
  wires:
  roll_control/1 -> roll_cmd/1
  Demux4/3 -> pitch_control/4
  Demux4/2 -> pitch_control/3
  Demux4/1 -> pitch_control/2
  pitch_params/1 -> Demux4/1
  Demux3/3 -> roll_control/4
  Demux3/2 -> roll_control/3
  Demux3/1 -> roll_control/2
  pitch_control/1 -> Gain/1
  e_roll/1 -> roll_control/1
  e_pitch/1 -> pitch_control/1
  roll_params/1 -> Demux3/1
  Gain/1 -> pitch_cmd/1

== matlab function Bixler_withAutoPilot/MATLAB Function1 ==
  data: u input uint16; y output uint16
function y = invertpwm(u)

y = uint16(1500-(single(u)-1500));

== matlab function Bixler_withAutoPilot/MATLAB Function ==
  data: u input uint16; y output uint16
function y = invertpwm(u)

y = uint16(1500-(single(u)-1500));

== matlab function Bixler_withAutoPilot/MATLAB Function2 ==
  data: signals input uint16; y output single
function y = pwm2signal(signals)

y = single(signals);
% Shift to center
y = y-1500;
% Range is ~1000-2000, ie +-500, but in is +-1
y = y./500;

== matlab function Bixler_withAutoPilot/MATLAB Function3 ==
  data: signals input; y output uint16
function y = signal2pwm(signals)

y = zeros(size(signals)); % y is hard set to uint16


% Range is ~1000-2000, ie +-500, but in is +-1
signals = signals.*500;
% Shift to center PWM
signals = signals+1500;
y = uint16(signals);

== matlab function Bixler_withAutoPilot/MATLAB Function4 ==
  data: switcher input uint16; pP output single; adjuster input uint16; pI output single; pD output single; enabler input uint16; ControlSelector input uint16; rP output single; rI output single; rD output single
function [pP,pI,pD,rP,rI,rD] = fcn(switcher, adjuster, enabler, ControlSelector)

persistent pkP pkI pkD rkP rkI rkD;
if isempty(pkP)
    pkP = single(1);
end
if isempty(pkI)
    pkI = single(0.4);
end
if isempty(pkD)
    pkD = single(0.025);
end
if isempty(rkP)
    rkP = single(1);
end
if isempty(rkI)
    rkI = single(0.4);
end
if isempty(rkD)
    rkD = single(0.05);
end

if enabler>1500
    if ControlSelector < 1400 % Top, Roll controll
        if switcher < 1400 % Top, P
            rkP = 1+(single(adjuster)-1500)./500; 
        elseif switcher > 1600 % Bottom, D
            rkD = 0.05+0.05*(single(adjuster)-1500)./500;
        else
            rkI = 0.4+0.4*(single(adjuster)-1500)./500;
        end
    elseif ControlSelector < 1600 % Mid, Pitch control
        if switcher < 1400 % Top, P
            pkP = 1+(single(adjuster)-1500)./500; 
        elseif switcher > 1600 % Bottom, D
            pkD = 0.025+0.025*(single(adjuster)-1500)./500;
        else
            pkI = 0.4+0.4*(single(adjuster)-1500)./500;
        end
    else
        % No controller set here yet
    end
end

pP = pkP;
pI = pkI;
pD = pkD;
rP = rkP;
rI = rkI;
rD = rkD;

== matlab function Bixler_withAutoPilot/ModeSelector ==
  data: selector input uint16; cmds output uint16 size=[2,1]; manual_cmds input uint16; FBW_cmds input uint16; enableFBW output boolean; enableAuto output; auto_cmds input
function [cmds,enableFBW,enableAuto] = fcn(selector, manual_cmds, FBW_cmds, auto_cmds)

if selector>1600 % Auto mode, stick down on remote
    cmds = auto_cmds;
    enableFBW = false;
    enableAuto = true;
elseif selector>1400% Midpoint, as I flew at MUST first time
    cmds = FBW_cmds;
    enableFBW = true;
    enableAuto = false;
else
    cmds = manual_cmds; % As midpoint, but less pitch sensitive.
    enableFBW = false;
    enableAuto = false;
end

== matlab function Bixler_withAutoPilot/MATLAB Function10 ==
  data: signals input; y output uint16
function y = signal2pwm(signals)

y = zeros(size(signals)); % y is hard set to uint16


% Range is ~1000-2000, ie +-500, but in is +-1
signals = signals.*500;
% Shift to center PWM
signals = signals+1500;
y = uint16(signals);

== matlab function Bixler_withAutoPilot/linegenerator ==
  settings: updateMethod=DISCRETE
  data: r input single; rspeed output single; wpN output single; dist2wp output single; linevec output single; vec2line output single; wp_r output single; waypoints input single; numwp input single
function [rspeed,wpN, dist2wp, linevec, vec2line, wp_r] = LineGenerator( r, waypoints, numwp)

% Keep track of which waypoint we are going to
persistent waypointno;
persistent wp;
persistent wp_prev;
if isempty(waypointno)
    waypointno=single(2);
    wp=waypoints(waypointno,:)';
    wp_prev=waypoints(waypointno-1,:)';
end

%initialize variables
rspeed = single(0);
vec2line = single([0,0,0])';

% if current waypoint is the start wp/home wp jump immediately to next.
dist2wp = sqrt( sum( (wp(1:3)-r).^2 ) );
if dist2wp <= wp(5)
    if waypointno < numwp
        waypointno = waypointno+1;
    else
        waypointno = single(1); % 
    end
    wp_prev = wp;
    wp = waypoints(waypointno,:)';
end
rspeed = wp(4);
wp_r = wp(1:3); % Next waypoint position, v has been scaled away thus wp_r

% find vector between last waypoint and current target
linevec = (wp(1:3)-wp_prev(1:3))./sqrt( sum((wp(1:3)-wp_prev(1:3)).^2) );

if  dot(linevec, wp(1:3)-r) < 0 
    linevec(1:3)=-linevec(1:3);
end

a = wp_prev(1:3);               % Points to "start of line"
n = linevec;                    % Points toward next wp
vec2line = a-r - dot(a-r,n)*n;  % Points toward closest point on line
wpN = waypointno;

== matlab function Bixler_withAutoPilot/PX4 SD Card Logger/SDCard_logger ==
  data: en input boolean; data input; logname parameter uint8; cacheflag parameter boolean; numRecs parameter uint32
%% PX4 SD Card Logger
% Note: All data needs to be of the same type (e.g. double)
% Header information format:
%           String "MWLOG"
%           Time/Date 4 bytes (time())
%           Number of Signals per record Logged 1 byte (256 max)
%           Data Type of Signals Logged  1 byte (1-10)
%           Number of bytes per record 2 bytes (65535 max)
% This does NOT include the number of data sets logged.
% i.e. The Reader is responsible for reading until EOF.
% Steve Kuznicki
% Copyright 2018 The MathWorks, Inc.

function SDCard_logger(en, data, logname, cacheflag, numRecs)

persistent fp isflushed isopen count  elem_size vect_size datastore timestore count_prev

if coder.target('Rtw')
    
    coder.cinclude('<stdio.h>');
    coder.cinclude('<time.h>');
    
    if coder.target('Rtw')
        coder.cinclude('<drivers/drv_hrt.h>');
    end
    
    if coder.target('Rtw')
        timestamp=coder.opaque('uint64_t');
        timestamp=coder.ceval('hrt_absolute_time');
    else
        timestamp = uint64(0);
    end
    
    if isempty(count)
        count = uint32(0);
        count_prev=count;
        fp = coder.opaque('FILE*', 'NULL');
        isflushed = false;
        if cacheflag == true
            datastore = zeros(numRecs*uint32(coder.const(numel(data))), 1, 'like', data);
            timestore=uint64(zeros(numRecs, 1));
        end
        
        [elsize, eltype] = get_elem_size(data);
        elem_size = coder.const(uint16(elsize));
        elem_type = coder.const(uint8(eltype));
        vect_size = coder.const(uint8(numel(data)));
        coder.ceval('printf',['OPENING file %s vect_size %d elem_size %d numRecs %d %c' uint8(0)], ...
            [logname,'.bin', int8(0)], uint32(vect_size), uint32(elem_size), uint32(numRecs), uint8(10));
        fp = coder.ceval('fopen', [logname,'.bin', int8(0)], ['wb', int8(0)]);
        isopen = true;
        
        % Write header information here
        % header token + version
        mlStrVer = 'MWLOG';
        coder.ceval('fwrite', coder.rref(mlStrVer), uint32(1), length(mlStrVer), fp);
        % date/time
        tm = uint32(0);
        tmptr = uint32(0);
        tm = coder.ceval('time',coder.wref(tmptr));
        coder.ceval('fwrite', coder.rref(tm), uint32(4), uint32(1), fp);
        % number of elements in each record
        coder.ceval('fwrite', coder.rref(vect_size), uint32(1), uint32(1), fp);
        % data type of the elements
        coder.ceval('fwrite', coder.rref(elem_type), uint32(1), uint32(1), fp);
        % size of each record in bytes
        recSize = elem_size * uint16(vect_size);
        coder.ceval('fwrite', coder.rref(recSize), uint32(2), uint32(1), fp);
    end
    
    
    if (en && (count < numRecs))
        
        if isopen == false
            % open file in append mode
            fp = coder.ceval('fopen', [logname,'.bin', int8(0)], ['ab', int8(0)]);
            isflushed = false;
            isopen = true;
            count_prev=count;
        end
        
        % cache data in memory or use fwrite
        if cacheflag == true
            addr = (count*uint32(vect_size))+1;
            for idx = 1:vect_size
                datastore(addr) = data(idx);
                addr = addr + 1;
            end
            timestore(count+uint32(1))=uint64(timestamp);
        else
            coder.ceval('fwrite', coder.rref(data), elem_size, vect_size, fp);
            if coder.target('Rtw')
                coder.ceval('fwrite', coder.rref(timestamp), uint32(8), uint32(1), fp);
            end
        end
        count = count + uint32(1);
        
    else
        if isopen == true
            if ~isflushed
                coder.ceval('printf',['CLOSING file. count = %d %c' uint8(0)], uint32(count), uint8(10));
                if cacheflag
                    for idx=count_prev+1:count
                        for idx2=(idx-1)*double(vect_size)+1:(idx-1)*double(vect_size)+double(vect_size)
                            coder.ceval('fwrite', coder.rref(datastore(idx2)), elem_size, uint32(1), fp);
                        end
                        coder.ceval('fwrite', coder.rref(timestore(idx)), uint32(8), uint32(1), fp);
                    end
                end
                coder.ceval('fflush', fp);
                isflushed = true;
            end
            coder.ceval('fclose', fp);
        end
        isopen = false;
    end
end

% return the size of the element in bytes
    function [elem_size, dtype] = get_elem_size(data)
        switch(class(data))
            case 'double'
                elem_size = 8;
                dtype = 1;
            case 'single'
                elem_size = 4;
                dtype = 2;
            case 'int32'
                elem_size = 4;
                dtype = 3;
            case 'uint32'
                elem_size = 4;
                dtype = 4;
            case 'int16'
                elem_size = 2;
                dtype = 5;
            case 'uint16'
                elem_size = 2;
                dtype = 6;
            case 'int8'
                elem_size = 1;
                dtype = 7;
            case 'uint8'
                elem_size = 1;
                dtype = 8;
            case 'logical'
                elem_size = 1;
                dtype = 9;
            case 'embedded.fi'
                nt = numerictype(data);
                elem_size = 2^ceil(log2(ceil(nt.WordLength / 8)));
                dtype = 10;
        end
        if ~isreal(data)
            elem_size = elem_size*2;
        end
        
        elem_size = uint16(elem_size);
        dtype = uint8(dtype);
    end
end
